simulink model "sm_car_testrig_liveaxle"  (R2020b)
settings: Solver=VariableStepAuto  StartTime=0.0  StopTime=10.0  RelTol=1e-3  EnableMultiTasking=on
libraries: fl_lib x6, sm_car_lib x4, sm_lib x4, Susp_LiveAxle x1, nesl_utility x1
Description:
  | Copyright 2020 The MathWorks, Inc.
settings Model: Creator=smiller  LastModifiedBy=smiller
settings DataIOCC: LimitDataPoints=on  ReturnWorkspaceOutputs=off
settings OptimizationCC: LifeSpan=inf
settings DebuggingCC: AllowSymbolicDim=off  SFUnexpectedBacktrackingDiag=warning  SFNoUnconditionalDefaultTransitionDiag=warning  SFExecutionAtInitializationDiag=none  ArithmeticOperatorsInVariantConditions=warning
settings SFSimCC: SimUseLocalCustomCode=off  CustomCodeUndefinedFunction=UseInterfaceOnly
settings RTWCC: RTWUseLocalCustomCode=off
settings CodeAppCC: StateflowObjectComments=on
settings GRTTargetCC: TargetLangStandard=C89/C90 (ANSI)
settings ConfigComp: CovMetricSettings=dw  CovSaveCumulativeToWorkspaceVar=on  CovSaveSingleToWorkspaceVar=on  CovExternalEMLEnable=off  CovSFcnEnable=off
settings SimscapeCC: SimscapeNominalValues="[{\"value\":\"10\",\"unit\":\"V\"},{\"value\":\"1\",\"unit\":\"A\"},{\"value\":\"10\",\"unit\":\"N*m\"},{\"value\":\"10\",\"unit\":\"bar\"},{\"value\":\"100\",\"unit\":\"kJ/kg\"},{\"value\":\"1\",\"unit\":\"kW\"},{\"value\":\"300\",\"unit\":\"K\"},{\"value\":\"100\",\"unit\":\"cm^3/s\"},{\"value\":\"1\",\"unit\":\"kN\"},{\"value\":\"1\",\"unit\":\"g/cm^3\"},{\"value\":\"1\",\"unit\":\"l\"},{\"value\":\"1\",\"unit\":\"cm^2\"},{\"value\":\"60\",\"unit\":\"Hz\"}]"  SimscapeLogType=all  SimscapeLogDataHistory=10000
settings ConfigurationSet: Description=SimMechanics 2G
settings ExplorerConfigSet: InternalSimMechanicsExplorerSettings="<ExplorerConfiguration><canonicalview>default</canonicalview><AnimationSetting><BasePlaybackSpeed>1.0</BasePlaybackSpeed><PlaybackSpeedFactor>1.0</PlaybackSpeedFactor></AnimationSetting><TilePanel><TileInfo><Tiles Columns=\"1\" Count=\"1\" Rows=\"1\"><Column Weight=\"1\"/><Row Weight=\"1\"/><Tile Height=\"1\" Width=\"1\" X=\"0\" Y=\"0\"/></Tiles></TileInfo><SceneInfo><SceneViewer><BGColor><R>1</R><G>1</G><B>1</B></BGColor><Camera><DoPerspective>off</DoPerspective><Position><X>0.715338968235045503</X><Y>-0.688588974648837282</Y><Z>1.00196398340167869</Z></Position><Center><X>0.0133749413552901181</X><Y>0.0133750522309180331</Y><Z>0.29999995652192335</Z></Center><Up><X>-0.408248290463863073</X><Y>0.408248290463863073</Y><Z>0.816496580927726145</Z></Up><ViewLimDist>1</ViewLimDist><YLim>0.730190855860710197</YLim><XLim>0.978455746853351682</XLim></Camera></SceneViewer></SceneInfo></TilePanel><MechEditorPanel><Cameras/><GfxPanelCameraMap/><VideoCreator><PlaybackSpeedRatio>1.0</PlaybackSpeedRatio><FrameRate>30</FrameRate><VideoFormat>Motion JPEG AVI</VideoFormat><FrameSize>auto</FrameSize></VideoCreator></MechEditorPanel></ExplorerConfiguration>"

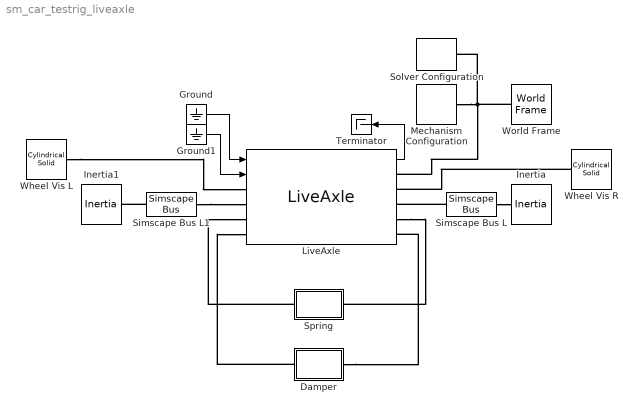
== system sm_car_testrig_liveaxle ==
  Damper : Subsystem
  Ground : Ground
  Ground1 : Ground
  Inertia : fl_lib/Mechanical/Rotational Elements/Inertia  inertia=0.01 kg*m^2  num_ports=foundation.enum.numPorts2.one  w_specify=on  w_priority=None  w=0 rad/s  w_nominal_specify=off  w_nominal_unit=rad/s  w_nominal_value=1  t_specify=off  t_priority=None  t=0 N*m  t_nominal_specify=off  t_nominal_unit=N*m  t_nominal_value=1
  Inertia1 : fl_lib/Mechanical/Rotational Elements/Inertia  inertia=0.01 kg*m^2  num_ports=foundation.enum.numPorts2.one  w_specify=on  w_priority=None  w=0 rad/s  w_nominal_specify=off  w_nominal_unit=rad/s  w_nominal_value=1  t_specify=off  t_priority=None  t=0 N*m  t_nominal_specify=off  t_nominal_unit=N*m  t_nominal_value=1
  LiveAxle : Susp_LiveAxle/LiveAxle  VariantControl=LiveAxle  Init=Init.Rear  hp_shock_top=Vehicle.Chassis.SuspR.LiveAxle.Shock.sTop.Value  hp_shock_bot=Vehicle.Chassis.SuspR.LiveAxle.Shock.sBottom.Value  hp_leaf_body=Vehicle.Chassis.SuspR.LiveAxle.Leaf.sBody.Value  hp_leaf_axle=Vehicle.Chassis.SuspR.LiveAxle.Leaf.sAxle.Value  hp_whl_ctr=Vehicle.Chassis.SuspR.LiveAxle.sWheelCentre.Value  axle_rad=Vehicle.Chassis.SuspR.LiveAxle.Axle.radius.Value  axle_mass=Vehicle.Chassis.SuspR.LiveAxle.Axle.m.Value  leaf_w=Vehicle.Chassis.SuspR.LiveAxle.Leaf.xWidth.Value  leaf_t=Vehicle.Chassis.SuspR.LiveAxle.Leaf.xThickness.Value  leaf_rho=Vehicle.Chassis.SuspR.LiveAxle.Leaf.density.Value  leaf_E=Vehicle.Chassis.SuspR.LiveAxle.Leaf.E.Value  leaf_nu=Vehicle.Chassis.SuspR.LiveAxle.Leaf.nu.Value  leaf_zeta=Vehicle.Chassis.SuspR.LiveAxle.Leaf.zDamping.Value  piston_mass=Vehicle.Chassis.SuspR.LiveAxle.Shock.mPiston.Value  cyl_mass=Vehicle.Chassis.SuspR.LiveAxle.Shock.mCylinder.Value  shock_xmax=Vehicle.Chassis.SuspR.LiveAxle.Endstop.xMax.Value  shock_xmin=Vehicle.Chassis.SuspR.LiveAxle.Endstop.xMin.Value
  Mechanism Configuration : sm_lib/Utilities/Mechanism Configuration  UniformGravity=Constant  GravityVector=[0 0 -9.80665]  GravityVectorUnits=m/s^2  GravityUnits=m/s^2  LinearizationDelta=0.001  JointModeTransitionNonlinearIterations=2
  Simscape Bus L : SimscapeBus  HierarchyStrings=Axle1D
  Simscape Bus L1 : SimscapeBus  HierarchyStrings=Axle1D
  Solver Configuration : nesl_utility/Solver Configuration  PhysicalDomain=network_engine_domain  SubClassName=solver  LeftPortType=input  RightPortType=generic  Tones=[]  Harmonics=[]  SimulateNoise=off  Profile=off  UseLocalSampling=off  EnableSwitchedLinearOptims=on  FrequencyDomain=off  UseCCode=off  RelTol=0.001  AbsTol=1e-06  MinStep=1e-09  ToWorkspace=off  RevertToSquareIcSolve=off  NumHomotopyIterations=100  PhasorMode=off  PhasorModeNumHarmonics=1  DoDC=off  ResidualTolerance=1e-09  UseLocalSolver=off  LocalSolverChoice=NE_BACKWARD_EULER_ADVANCER  LocalSolverSampleTime=0.001  DoFixedCost=off  MaxNonlinIter=3  MaxModeIter=2  ComputeImpulses=off  ImpulseIterations=2  LinearAlgebra=Sparse  EquationFormulation=NE_TIME_EF  DelaysMemoryBudget=1024  AutomaticFiltering=on  FilteringTimeConstant=0.001  PartitionStorageMethod=AS_NEEDED  PartitionMemoryBudget=1024  PartitionMethod=FAST
  Spring : Subsystem
  Terminator : Terminator
  Wheel Vis L : sm_lib/Body Elements/Cylindrical Solid  GraphicAmbientColor=[0.15 0.15 0.15 1.0]  BasedOnType=Density  CenterOfMass=[0 0 0]  CenterOfMassUnits=m  GraphicDiffuseColor=[0.5 0.5 0.5]  CylinderLength=0.1  CylinderLengthUnits=m  CylinderRadius=0.3  CylinderRadiusUnits=m  Density=1000  DensityUnits=kg/m^3  DoExposeReferenceFrame=on  GraphicEmissiveColor=[0.0 0.0 0.0 1.0]  ExportEntireGeometry=off  SerializedFrames=<Frames/>  MarkerShape=Sphere  MarkerSize=10  GraphicType=FromGeometry  InertiaType=CalculateFromGeometry  Mass=1  MassUnits=kg  MomentsOfInertia=[1 1 1]  MomentsOfInertiaUnits=kg*m^2  GraphicOpacity=0.3  ProductsOfInertia=[0 0 0]  ProductsOfInertiaUnits=kg*m^2  GraphicShininess=75  GraphicSpecularColor=[0.5 0.5 0.5 1.0]  GraphicVisPropType=SimpleVisualProperties
  Wheel Vis R : sm_lib/Body Elements/Cylindrical Solid  GraphicAmbientColor=[0.15 0.15 0.15 1.0]  BasedOnType=Density  CenterOfMass=[0 0 0]  CenterOfMassUnits=m  GraphicDiffuseColor=[0.5 0.5 0.5]  CylinderLength=0.1  CylinderLengthUnits=m  CylinderRadius=0.3  CylinderRadiusUnits=m  Density=1000  DensityUnits=kg/m^3  DoExposeReferenceFrame=on  GraphicEmissiveColor=[0.0 0.0 0.0 1.0]  ExportEntireGeometry=off  SerializedFrames=<Frames/>  MarkerShape=Sphere  MarkerSize=10  GraphicType=FromGeometry  InertiaType=CalculateFromGeometry  Mass=1  MassUnits=kg  MomentsOfInertia=[1 1 1]  MomentsOfInertiaUnits=kg*m^2  GraphicOpacity=0.3  ProductsOfInertia=[0 0 0]  ProductsOfInertiaUnits=kg*m^2  GraphicShininess=75  GraphicSpecularColor=[0.5 0.5 0.5 1.0]  GraphicVisPropType=SimpleVisualProperties
  World Frame : sm_lib/Frames and Transforms/World Frame
  wires:
  Ground/1 -> LiveAxle/1
  Ground1/1 -> LiveAxle/2
  LiveAxle/1 -> Terminator/1
  connections:
  Mechanism Configuration/RConn1 -- Solver Configuration/RConn1 -- World Frame/RConn1 -- LiveAxle/RConn1
  Wheel Vis L/RConn1 -- LiveAxle/LConn1
  Simscape Bus L/LConn1 -- Inertia/LConn1
  Spring/LConn1 -- LiveAxle/LConn3
  LiveAxle/RConn4 -- Spring/RConn1
  Simscape Bus L/RConn1 -- LiveAxle/RConn3
  Simscape Bus L1/LConn1 -- Inertia1/LConn1
  Simscape Bus L1/RConn1 -- LiveAxle/LConn2
  Damper/LConn1 -- LiveAxle/LConn4
  Wheel Vis R/RConn1 -- LiveAxle/RConn2
  Damper/RConn1 -- LiveAxle/RConn5

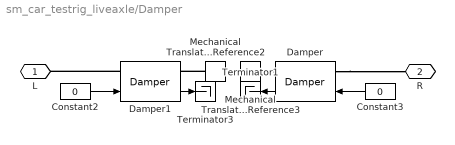
== system sm_car_testrig_liveaxle/Damper ==
  Constant2 : Constant  Value=0
  Constant3 : Constant  Value=0
  Damper : sm_car_lib/Springs Dampers/Damper  VariantControl=Variant1  LabelModeActiveChoice=Linear  Damper=Vehicle.Chassis.Damper.Rear  VariantLabel=Vehicle.Chassis.Damper.Rear.class.Value  InitTriggerDropdown=1
      settings: AttributesFormatString=%<ActiveVariant>
  Damper1 : sm_car_lib/Springs Dampers/Damper  VariantControl=Variant1  LabelModeActiveChoice=Linear  Damper=Vehicle.Chassis.Damper.Rear  VariantLabel=Vehicle.Chassis.Damper.Rear.class.Value  InitTriggerDropdown=1
      settings: AttributesFormatString=%<ActiveVariant>
  Mechanical Translational Reference2 : fl_lib/Mechanical/Translational Elements/Mechanical Translational Reference
  Mechanical Translational Reference3 : fl_lib/Mechanical/Translational Elements/Mechanical Translational Reference
  Terminator1 : Terminator
  Terminator3 : Terminator
  L : PMIOPort  Side=Left
  R : PMIOPort  Port=2  Side=Right
  wires:
  Damper/1 -> Terminator1/1
  Constant3/1 -> Damper/1
  Constant2/1 -> Damper1/1
  Damper1/1 -> Terminator3/1
  connections:
  Damper1/LConn1 -- L/RConn1
  Mechanical Translational Reference2/LConn1 -- Damper1/RConn1
  Mechanical Translational Reference3/LConn1 -- Damper/RConn1
  Damper/LConn1 -- R/RConn1

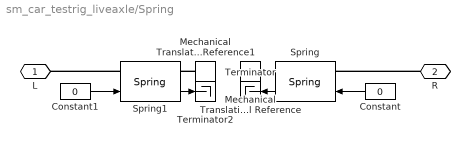
== system sm_car_testrig_liveaxle/Spring ==
  Constant : Constant  Value=0
  Constant1 : Constant  Value=0
  Mechanical Translational Reference : fl_lib/Mechanical/Translational Elements/Mechanical Translational Reference
  Mechanical Translational Reference1 : fl_lib/Mechanical/Translational Elements/Mechanical Translational Reference
  Spring : sm_car_lib/Springs Dampers/Spring  VariantControl=Variant1  LabelModeActiveChoice=Linear  Spring=Vehicle.Chassis.Spring.Front  VariantLabel=Vehicle.Chassis.Spring.Front.class.Value  InitTriggerDropdown=1
      settings: AttributesFormatString=%<ActiveVariant>
  Spring1 : sm_car_lib/Springs Dampers/Spring  VariantControl=Variant1  LabelModeActiveChoice=Linear  Spring=Vehicle.Chassis.Spring.Front  VariantLabel=Vehicle.Chassis.Spring.Front.class.Value  InitTriggerDropdown=1
      settings: AttributesFormatString=%<ActiveVariant>
  Terminator : Terminator
  Terminator2 : Terminator
  L : PMIOPort  Side=Left
  R : PMIOPort  Port=2  Side=Right
  wires:
  Spring1/1 -> Terminator2/1
  Constant1/1 -> Spring1/1
  Spring/1 -> Terminator/1
  Constant/1 -> Spring/1
  connections:
  Mechanical Translational Reference1/LConn1 -- Spring1/RConn1
  Mechanical Translational Reference/LConn1 -- Spring/RConn1
  R/RConn1 -- Spring/LConn1
  Spring1/LConn1 -- L/RConn1
